simulink model "mambo_offline_simulator"  (R2022b)
settings: Solver=VariableStepAuto  StartTime=0.0  StopTime=45  RelTol=1e-3
values from neighbouring files (symbols this model uses):
  A_angles = sysd_angles.den    [parrot_mambo_main.m]
  A_thrust = sysd_thrust.den    [parrot_mambo_main.m]
  angle_sat = 0.22    [parrot_mambo_main.m]
  B_angles = sysd_angles.num    [parrot_mambo_main.m]
  B_thrust = sysd_thrust.num    [parrot_mambo_main.m]
  delay = 0.08    [parrot_mambo_main.m]
  g = 9.81    [parrot_mambo_main.m]
  GLOBAL_PARAMETERS = [Ts m g Kv]    [parrot_mambo_main.m]
  initial_pos_conditions_M1 = [0 0 0]    [parrot_mambo_main.m]
  K_gain_lin = lqr(A, B, Q_gain_lin, R_gain_lin)    [parrot_mambo_main.m]
  Ki_x = 0.04    [parrot_mambo_main.m]
  Ki_y = 0.04    [parrot_mambo_main.m]
  Ki_z = 0.023    [parrot_mambo_main.m]
  m = 0.075    [parrot_mambo_main.m]
  phi_biais = 0.005    [parrot_mambo_main.m]
  sat_z = 1    [parrot_mambo_main.m]
  theta_biais = 0.005    [parrot_mambo_main.m]
  Tmax = 1.0088    [parrot_mambo_main.m]
  Tmin = 0.4786    [parrot_mambo_main.m]
  Ts = 0.01    [parrot_mambo_main.m]
  variance_boucle_attitude = 1e-7    (= 1e-07)    [parrot_mambo_main.m]
  variance_qualysis = 1e-6    (= 1e-06)    [parrot_mambo_main.m]
  x0 = -1.18    [parrot_mambo_main.m]
  y0 = -1.21    [parrot_mambo_main.m]
  z0 = 0.8    [parrot_mambo_main.m]
libraries: simulink x2, slpidlib x1
settings Model: Creator=susbielp  LastModifiedBy=phatdo
settings SolverCC: AlgebraicLoopSolver=TrustRegion
settings DataIOCC: ReturnWorkspaceOutputs=off
settings DebuggingCC: UnconnectedInputMsg=warning  UnconnectedOutputMsg=warning  UnconnectedLineMsg=warning  ArithmeticOperatorsInVariantConditions=warning
settings ModelReferenceCC: EnableRefExpFcnMdlSchedulingChecks=on
settings SFSimCC: CustomCodeUndefinedFunction=UseInterfaceOnly
settings RTWCC: DLArmComputeVersion=19.05

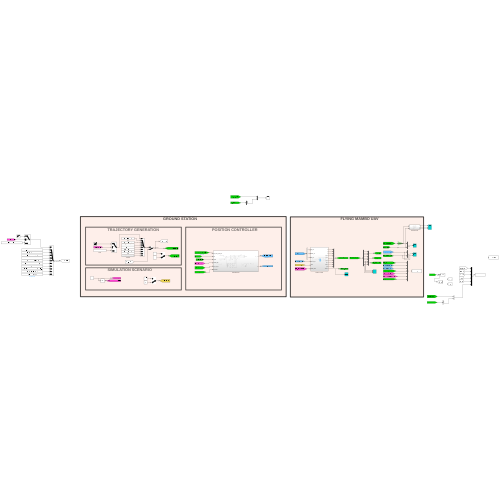
[thumbnail: Simulink's stored preview of the top-level diagram]
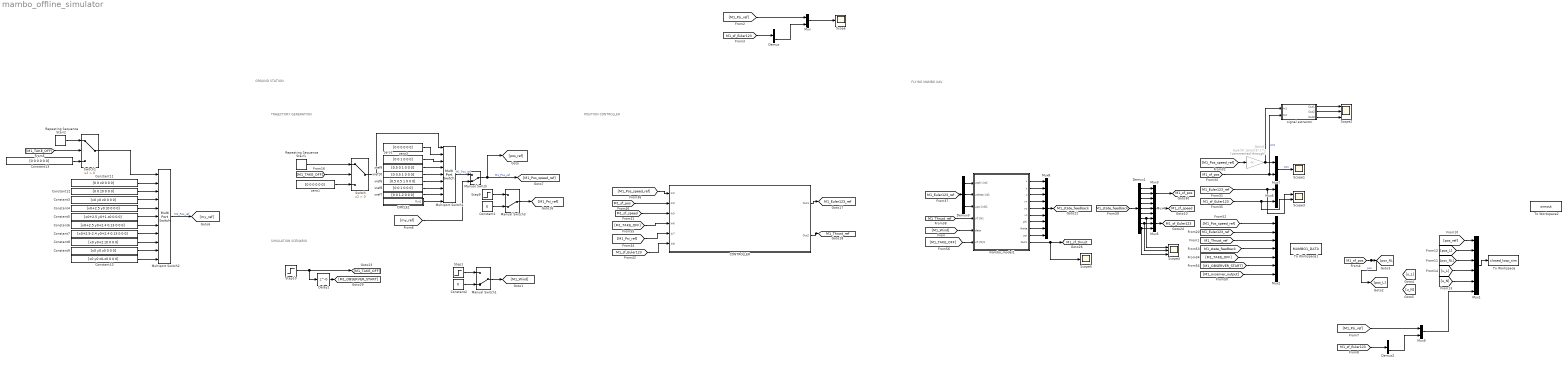
== system mambo_offline_simulator ==
  note: FLYING MAMBO UAV
  note: POSITION CONTROLLER
  note: TRAJECTORY GENERATION
  note: SIMULATION SCENARIO
  note: GROUND STATION
  CIRCLE1 : Subsystem
  CONTROLLER : Subsystem
  Constant1 : Constant  Value=0  OutDataTypeStr=double
  Constant10 : Constant  Value=[x0 y0 z0-z0 0 0 0]
  Constant11 : Constant  Value=[0 0 z0 0 0 0]
  Constant12 : Constant  Value=[0 0 z0 0 0 0]
  Constant13 : Constant  Value=[0 0 0 0 0 0]
  Constant2 : Constant  Value=0  OutDataTypeStr=double
  Constant3 : Constant  Value=[x0 y0 z0 0 0 0]
  Constant4 : Constant  Value=[x0+2.5 y0 z0 0 0 0]
  Constant5 : Constant  Value=[x0+2.5 y0+1 z0 0 0 0]
  Constant6 : Constant  Value=[x0+2.5 y0+2.4 0.13 0 0 0]
  Constant7 : Constant  Value=[x0+2.5-2.4 y0+2.4 0.13 0 0 0]
  Constant8 : Constant  Value=[x0 y0+2 z0 0 0 0]
  Constant9 : Constant  Value=[x0 y0 z0 0 0 0]
  Delay1 : Delay  DelayLength=0
  Demux : Demux  Outputs=3
  Demux1 : Demux  Outputs=9
  Demux2 : Demux  Outputs=3
  Demux3 : Demux  Outputs=3
  Gain4 : Gain  Commented=through  Gain=[eye(3) zeros(3) ]  Multiplication=Matrix(K*u) (u vector)
  Manual Switch : ManualSwitch  CurrentSetting=0
  Manual Switch1 : ManualSwitch  CurrentSetting=0
  Manual Switch3 : ManualSwitch  CurrentSetting=0
  Multiport Switch1 : MultiPortSwitch  DataPortOrder=Zero-based contiguous  Inputs=8  zeroidx=on  SaturateOnIntegerOverflow=off  InputSameDT=off
  Multiport Switch2 : MultiPortSwitch  DataPortOrder=Zero-based contiguous  Inputs=10  zeroidx=on  SaturateOnIntegerOverflow=off  InputSameDT=off
  Mux{,6..7,9} (4 alike) : Mux  Inputs=2
  Mux1 : Mux  Inputs=6
  Mux2 : Mux  Inputs=7
  Mux3 : Mux  Inputs=3
  Mux4 : Mux  Inputs=3
  Mux5 : Mux  Inputs=3
  Mux8 : Mux  Inputs=9
  Repeating Sequence Stair1 : simulink/Sources/Repeating Sequence Stair  OutValues=[1 2 1 3 1 4 1 6 7].'  tsamp=10  OutMin=[]  OutMax=[]  OutDataTypeStr=double  OutputDataTypeScalingMode=double  OutDataType=fixdt(0,8)  ConRadixGroup=Best Precision: Vector-wise  OutScaling=2^-12
  Repeating Sequence Stair2 : simulink/Sources/Repeating Sequence Stair  OutValues=[1 2 3 4 5 6 7 8 9].'  tsamp=task_ped  OutMin=[]  OutMax=[]  OutDataTypeStr=double  OutputDataTypeScalingMode=double  OutDataType=fixdt(0,8)  ConRadixGroup=Best Precision: Vector-wise  OutScaling=2^-12
  Scope : Scope
  Scope1 : Scope
  Scope2 : Scope  NumInputPorts=3
  Scope3 : Scope  NumInputPorts=2
  Scope4 : Scope  NumInputPorts=3
  Scope5 : Scope
  Step1 : Step  Time=20  Before=[0 0 0]  After=[2 0 0]  SampleTime=0
  Step10 : Step  Time=2  SampleTime=0
  Step9 : Step  Time=25  After=pi/2  SampleTime=0
  Switch : Switch  Criteria=u2 > Threshold  SaturateOnIntegerOverflow=off  InputSameDT=off
  Switch1 : Switch  Criteria=u2 > Threshold  SaturateOnIntegerOverflow=off  InputSameDT=off
  To Workspace : ToWorkspace  VariableName=closed_loop_sim  SaveFormat=Timeseries  SampleTime=-1
  To Workspace1 : ToWorkspace  VariableName=MAMBO1_DATA  SaveFormat=Timeseries  SampleTime=-1
  To Workspace2 : ToWorkspace  VariableName=simout  SaveFormat=Timeseries  SampleTime=-1
  mambo_model1 : Subsystem
  signal extractor : Subsystem
  xref10 : Constant  Value=[0 0.5 1 0 0 0]  OutDataTypeStr=double
  xref6 : Constant  Value=[0.5 0.5 1 0 0 0]  OutDataTypeStr=double
  xref7 : Constant  Value=[0 0 1.2 0 0 0]  OutDataTypeStr=double
  xref8 : Constant  Value=[0 0 1 0 0 0]  OutDataTypeStr=double
  xref9 : Constant  Value=[0.5 0 1 0 0 0]  OutDataTypeStr=double
  zero1 : Constant  Value=[0 0 0 0 0 0]  OutDataTypeStr=double
  zero2 : Constant  Value=[0 0 1 0 0 0]  OutDataTypeStr=double
  zero3 : Constant  Value=[0 0 0 0 0 0]  OutDataTypeStr=double
  tag scope: M1_Euler123_ref=global, M1_Thrust_ref=global, M1_sf_Euler123=global, M1_sf_pos=global, M1_sf_speed=global, M1_sf_thrust=global, M1_state_feedback=global
  wires:
  Mux5/1 -> [M1_sf_Euler123]
  Demux1/4 -> Mux4/1
  Demux1/1 -> Mux3/1
  Demux1/3 -> Mux3/3
  [M1_sf_pos] -> signal extractor/2(In2), Mux7/2  "pos"
  Mux7/1 -> Scope1/1  "pos"
  Demux1/6 -> Mux4/3
  [M1_OBSERVER_START] -> Mux2/6
  Demux1/5 -> Mux4/2
  [M1_sf_Euler123] -> Scope3/2, Mux6/2
  [M1_sf_speed] -> CONTROLLER/3(In5)
  [M1_Pos_speed_ref] -> CONTROLLER/1(In2)
  Demux1/2 -> Mux3/2
  Demux1/8 -> Scope4/2, Mux5/2
  Mux4/1 -> [M1_sf_speed]
  [M1_sf_pos] -> CONTROLLER/2(In3)
  [M1_Euler123_ref] -> Scope3/1, Mux6/1
  [M1_ovserver_output] -> Mux2/7
  [M1_Pos_speed_ref] -> Gain4/1
  [M1_TAKE_OFF] -> Mux2/5
  [M1_TAKE_OFF] -> CONTROLLER/4(In6)
  [M1_Euler123_ref] -> Mux2/2
  [M1_state_feedback] -> Demux1/1
  [M1_state_feedback] -> Mux2/4
  CONTROLLER/2(Out2) -> [M1_Thrust_ref]
  Mux3/1 -> [M1_sf_pos]
  CONTROLLER/1(Out1) -> [M1_Euler123_ref]
  Demux1/9 -> Scope4/3, Mux5/3
  [M1_Pos_speed_ref] -> Mux2/1
  Step10/1 -> Delay1/1, [M1_TAKE_OFF]
  Delay1/1 -> [M1_OBSERVER_START]
  CIRCLE1/1(Out1) -> Multiport Switch1/9
  zero3/1 -> Multiport Switch1/2
  Manual Switch/1 -> [pos_ref], [M1_Pos_speed_ref]  "M1_Pos_ref"
  xref8/1 -> Multiport Switch1/7
  xref7/1 -> Multiport Switch1/8
  xref9/1 -> Multiport Switch1/4
  xref10/1 -> Multiport Switch1/5
  zero2/1 -> Multiport Switch1/3
  xref6/1 -> Multiport Switch1/6
  Step9/1 -> Manual Switch3/1
  [M1_Thrust_ref] -> Mux2/3
  Manual Switch3/1 -> [M1_Psi_ref]
  Switch/1 -> Multiport Switch1/1
  [M1_TAKE_OFF] -> Switch/2
  zero1/1 -> Switch/3
  Repeating Sequence Stair1/1 -> Switch/1
  Constant1/1 -> Manual Switch3/2
  [M1_Euler123_ref] -> Demux3/1
  mambo_model1/6(vz) -> Mux8/6
  mambo_model1/8(theta) -> Mux8/8
  mambo_model1/7(phi) -> Mux8/7
  mambo_model1/5(vy) -> Mux8/5
  mambo_model1/9(psi) -> Mux8/9
  [M1_Thrust_ref] -> mambo_model1/4(uT [N])
  mambo_model1/4(vx) -> Mux8/4
  Demux3/2 -> mambo_model1/2(utheta [rd])
  Mux8/1 -> [M1_state_feedback]
  mambo_model1/10(Out1) -> Scope5/1, [M1_sf_thrust]
  mambo_model1/3(z) -> Mux8/3
  mambo_model1/2(y) -> Mux8/2
  Demux3/3 -> mambo_model1/3(upsi [rd]1)
  Demux3/1 -> mambo_model1/1(utphi [rd])
  [M1_TAKE_OFF] -> mambo_model1/6(uT [N]1)
  mambo_model1/1(x) -> Mux8/1
  [M1_Wind] -> mambo_model1/5(data)
  Step1/1 -> Manual Switch1/1
  Constant2/1 -> Manual Switch1/2
  Manual Switch1/1 -> [M1_Wind]
  Gain4/1 -> signal extractor/1(In1), Mux7/1
  signal extractor/1(Out1) -> Scope2/1
  signal extractor/2(Out2) -> Scope2/2
  signal extractor/3(Out3) -> Scope2/3
  [M1_sf_Euler123] -> Demux/1
  [M1_Psi_ref] -> Mux/1
  Demux/3 -> Mux/2
  Mux/1 -> Scope/1
  [pos_ref] -> Mux1/1
  Mux1/1 -> To Workspace/1
  [u_N] -> Mux1/5
  [pos_L] -> Mux1/2
  [pos_NL] -> Mux1/3
  [u_L] -> Mux1/4
  [M1_sf_pos] -> [pos_L], [pos_NL]  "pos"
  Repeating Sequence Stair2/1 -> Switch1/1
  [M1_TAKE_OFF] -> Switch1/2
  Switch1/1 -> Multiport Switch2/1
  Constant11/1 -> Multiport Switch2/2
  Constant13/1 -> Switch1/3
  Constant12/1 -> Multiport Switch2/3
  Multiport Switch1/1 -> Manual Switch/1  "M1_Pos_ref"
  Constant3/1 -> Multiport Switch2/4
  Constant4/1 -> Multiport Switch2/5
  Constant5/1 -> Multiport Switch2/6
  Constant6/1 -> Multiport Switch2/7
  Constant7/1 -> Multiport Switch2/8
  Constant8/1 -> Multiport Switch2/9
  Constant9/1 -> Multiport Switch2/10
  Multiport Switch2/1 -> [my_ref]  "M1_Pos_ref"
  [my_ref] -> Manual Switch/2
  [M1_Psi_ref] -> CONTROLLER/5(In7)
  [M1_sf_Euler123] -> CONTROLLER/6(In8)
  [M1_sf_Euler123] -> Demux2/1
  [M1_Psi_ref] -> Mux9/1
  Demux2/3 -> Mux9/2
  Mux9/1 -> Mux1/6
  Demux1/7 -> Scope4/1, Mux5/1
  Constant10/1 -> Multiport Switch2/11

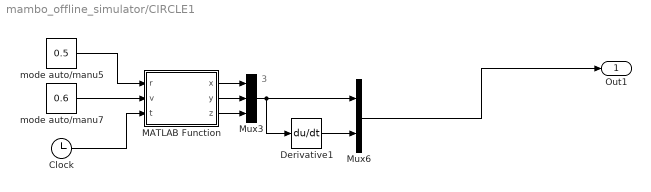
== system mambo_offline_simulator/CIRCLE1 ==
  note: 3
  Clock : Clock
  Derivative1 : Derivative  CoefficientInTFapproximation=4*Ts
  MATLAB Function : MATLAB Function  TreatAsAtomicUnit=on
  Mux3 : Mux  Inputs=3
  Mux6 : Mux  Inputs=2
  mode auto/manu5 : Constant  Value=0.5  OutDataTypeStr=double
  mode auto/manu7 : Constant  Value=0.6  OutDataTypeStr=double
  Out1 : Outport
  wires:
  MATLAB Function/2(y) -> Mux3/2
  Derivative1/1 -> Mux6/2
  Mux3/1 -> Mux6/1, Derivative1/1
  Mux6/1 -> Out1/1
  mode auto/manu5/1 -> MATLAB Function/1(r)
  Clock/1 -> MATLAB Function/3(t)
  MATLAB Function/1(x) -> Mux3/1
  mode auto/manu7/1 -> MATLAB Function/2(v)
  MATLAB Function/3(z) -> Mux3/3

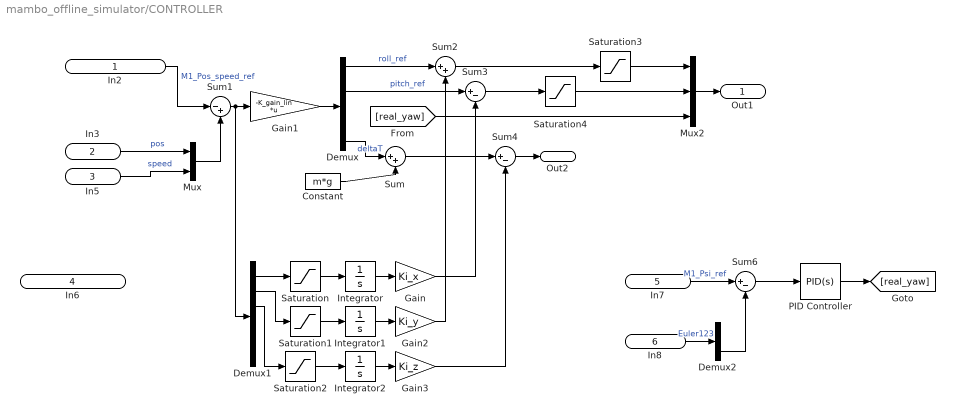
== system mambo_offline_simulator/CONTROLLER ==
  In2 : Inport
  In3 : Inport  Port=2
  In5 : Inport  Port=3
  In6 : Inport  Port=4
  In7 : Inport  Port=5
  In8 : Inport  Port=6
  Constant : Constant  Value=m*g
  Demux : Demux
  Demux1 : Demux  Outputs=6
  Demux2 : Demux  Outputs=3
  Gain : Gain  Gain=Ki_x
  Gain1 : Gain  Gain=-K_gain_lin  Multiplication=Matrix(K*u) (u vector)
  Gain2 : Gain  Gain=Ki_y
  Gain3 : Gain  Gain=Ki_z
  Integrator : Integrator
  Integrator1 : Integrator
  Integrator2 : Integrator
  Mux : Mux  Inputs=2
  Mux2 : Mux  Inputs=3
  PID Controller : slpidlib/PID Controller  Controller=PID  Form=Parallel  TimeDomain=Continuous-time  UseExternalTs=off  SampleTime=-1  IntegratorMethod=Forward Euler  FilterMethod=Forward Euler  ControllerParametersSource=internal  P=1.9  I=4.5  UseKiTs=off  D=0.05  N=8.8  UseFilter=on  TunerSelectOption=Transfer Function Based (PID Tuner App)  InitialConditionSource=internal  InitialConditionForIntegrator=0  InitialConditionForFilter=0  DifferentiatorICPrevScaledInput=0  ExternalReset=none  TrackingMode=off  Kt=1  LimitOutput=off  SatLimitsSource=internal  UpperSaturationLimit=inf  LowerSaturationLimit=-inf  LinearizeAsGain=on  AntiWindupMode=none  Kb=1  LimitIntegrator=off  UpperIntegratorSaturationLimit=inf  LowerIntegratorSaturationLimit=-inf  POutMin=[]  POutMax=[]  IOutMin=[]  IOutMax=[]  DOutMin=[]  DOutMax=[]  NOutMin=[]  NOutMax=[]  SumOutMin=[]  SumOutMax=[]  SaturationOutMin=[]  SaturationOutMax=[]  PParamMin=[]  PParamMax=[]  IParamMin=[]  IParamMax=[]  DParamMin=[]  DParamMax=[]  NParamMin=[]  NParamMax=[]  KbParamMin=[]  KbParamMax=[]  KtParamMin=[]  KtParamMax=[]  KbOutMin=[]  KbOutMax=[]  KtOutMin=[]  KtOutMax=[]  IntegratorOutMin=[]  IntegratorOutMax=[]  FilterOutMin=[]  FilterOutMax=[]  SumI1OutMin=[]  SumI1OutMax=[]  SumI2OutMin=[]  SumI2OutMax=[]  SumI3OutMin=[]  SumI3OutMax=[]  SumI4OutMin=[]  SumI4OutMax=[]  SumDOutMin=[]  SumDOutMax=[]  DifferentiatorOutMin=[]  DifferentiatorOutMax=[]  FilterDiffOutCoefMin=[]  FilterDiffOutCoefMax=[]  ReciprocalOutMin=[]  ReciprocalOutMax=[]  SumDenOutMin=[]  SumDenOutMax=[]  SumNumOutMin=[]  SumNumOutMax=[]  DivideOutMin=[]  DivideOutMax=[]  UdiffTsProdOutMin=[]  UdiffTsProdOutMax=[]  NTsProdOutMin=[]  NTsProdOutMax=[]  UintegralTsProdOutMin=[]  UintegralTsProdOutMax=[]  UngainTsProdOutMin=[]  UngainTsProdOutMax=[]  ClampingZeroOutDataTypeStr=Inherit: Inherit via back propagation  ClampingZeroOutMin=[]  ClampingZeroOutMax=[]  FilterDenConstantOutDataTypeStr=Inherit: Inherit via back propagation  FilterDenConstantOutMin=[]  FilterDenConstantOutMax=[]  PCopyOutDataTypeStr=Inherit: Inherit via back propagation  PCopyOutMin=[]  PCopyOutMax=[]  NCopyOutDataTypeStr=Inherit: Inherit via back propagation  NCopyOutMin=[]  NCopyOutMax=[]  IntegratorContinuousStateAttributes=''  IntegratorStateMustResolveToSignalObject=off  IntegratorRTWStateStorageClass=Auto  FilterContinuousStateAttributes=''  FilterStateMustResolveToSignalObject=off  FilterRTWStateStorageClass=Auto  ParallelPVariant=InternalParameters  IdealPVariant=Disabled  IVariant=InternalParameters  DVariant=InternalParameters  IntegratorVariant=Continuous  SatVariant=Disabled  AWVariant=Passthrough  PCopyVariant=Disabled  TRVariant=Disabled  FdbkBlocksVariant=Forward  IdealPFdbkVariant=Disabled  SatFdbkVariant=Disabled  DerivativeFilterVariant=ContFilter  NVariant=InternalParameters  NCopyVariant=Disabled  FilterICVariant=InternalICsFilter  IntegratorICVariant=InternalICs  ExternalResetVariant=Disabled  TRSumVariant=Passthrough  SumFdbkVariant=Disabled  SumVariant=Sum_PID  TsampFilterVariant=InternalTs  TsampNgainVariant=Passthrough  TsampIntegralVariant=Passthrough  ExternalSaturationOutDataTypeStr=Inherit: Same as second input
  Saturation : Saturate  UpperLimit=0.02  LowerLimit=-0.02
  Saturation1 : Saturate  UpperLimit=0.02  LowerLimit=-0.02
  Saturation2 : Saturate  UpperLimit=sat_z  LowerLimit=-sat_z
  Saturation3 : Saturate  UpperLimit=0.1  LowerLimit=-0.1
  Saturation4 : Saturate  UpperLimit=0.1  LowerLimit=-0.1
  Sum : Sum  Inputs=|++
  Sum1 : Sum  Inputs=|-+
  Sum2 : Sum  Inputs=|++
  Sum3 : Sum  Inputs=|+-
  Sum4 : Sum  Inputs=|+-
  Sum6 : Sum  Inputs=|+-
  Out1 : Outport
  Out2 : Outport  Port=2
  wires:
  Sum1/1 -> Demux1/1, Gain1/1
  In2/1 -> Sum1/1  "M1_Pos_speed_ref"
  Mux/1 -> Sum1/2
  Gain1/1 -> Demux/1
  In5/1 -> Mux/2  "speed"
  Mux2/1 -> Out1/1
  Constant/1 -> Sum/2
  Demux/4 -> Sum/1  "deltaT"
  In3/1 -> Mux/1  "pos"
  Demux1/3 -> Saturation2/1
  Demux1/1 -> Saturation/1
  Demux/1 -> Sum2/1  "roll_ref"
  Sum2/1 -> Saturation3/1
  Demux/2 -> Sum3/1  "pitch_ref"
  Sum3/1 -> Saturation4/1
  Sum4/1 -> Out2/1
  Sum/1 -> Sum4/1
  Integrator2/1 -> Gain3/1
  Gain/1 -> Sum3/2
  Gain2/1 -> Sum2/2
  Integrator/1 -> Gain/1
  Integrator1/1 -> Gain2/1
  Gain3/1 -> Sum4/2
  Saturation/1 -> Integrator/1
  Saturation1/1 -> Integrator1/1
  Demux1/2 -> Saturation1/1
  [real_yaw] -> Mux2/3
  In7/1 -> Sum6/1  "M1_Psi_ref"
  In8/1 -> Demux2/1  "Euler123"
  Sum6/1 -> PID Controller/1
  Demux2/3 -> Sum6/2
  PID Controller/1 -> [real_yaw]
  Saturation2/1 -> Integrator2/1
  Saturation3/1 -> Mux2/1
  Saturation4/1 -> Mux2/2

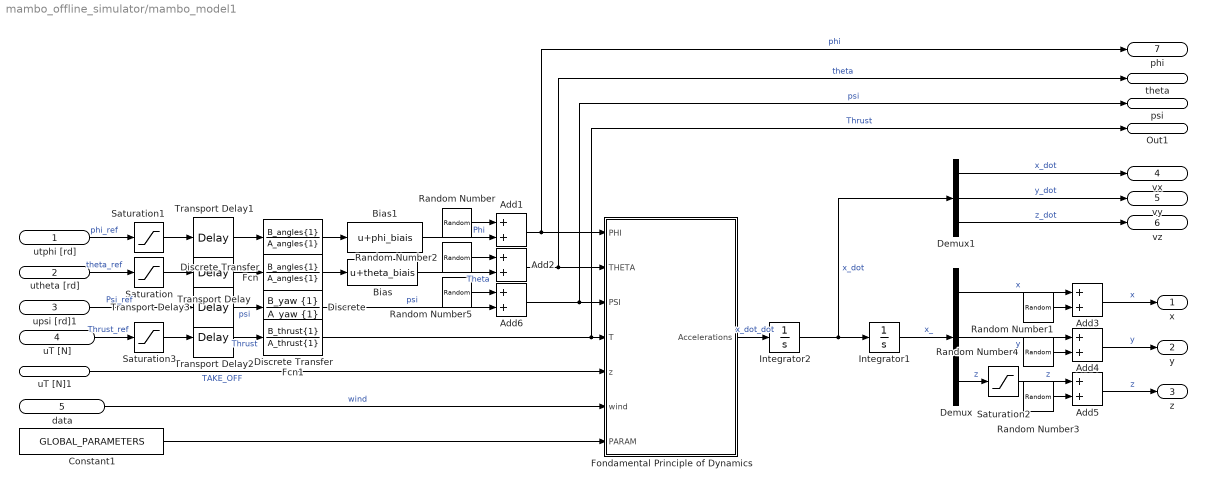
== system mambo_offline_simulator/mambo_model1 ==
  utphi [rd] : Inport
  utheta [rd] : Inport  Port=2
  upsi [rd]1 : Inport  Port=3
  uT [N] : Inport  Port=4
  data : Inport  Port=5
  uT [N]1 : Inport  Port=6
  " " : DiscreteTransferFcn  Numerator=B_angles{1}  Denominator=A_angles{1}  SampleTime=Ts
  Add{1..6} (6 alike) : Sum
  Bias : Bias  Bias=theta_biais  SaturateOnIntegerOverflow=off
  Bias1 : Bias  Bias=phi_biais  SaturateOnIntegerOverflow=off
  Constant1 : Constant  Value=GLOBAL_PARAMETERS
  Demux : Demux  Outputs=3
  Demux1 : Demux  Outputs=3
  "Discrete " : DiscreteTransferFcn  Numerator=B_yaw {1}  Denominator=A_yaw {1}  SampleTime=Ts
  Discrete Transfer Fcn : DiscreteTransferFcn  Numerator=B_angles{1}  Denominator=A_angles{1}  SampleTime=Ts
  Discrete Transfer Fcn1 : DiscreteTransferFcn  Numerator=B_thrust{1}  Denominator=A_thrust{1}  SampleTime=Ts
  Fondamental Principle of Dynamics : MATLAB Function  TreatAsAtomicUnit=on
  Integrator1 : Integrator  InitialCondition=initial_pos_conditions_M1
  Integrator2 : Integrator  InitialCondition=[0 0 0]
  Random Number : RandomNumber  Variance=variance_boucle_attitude  Seed=0.5  SampleTime=Ts
  Random Number1 : RandomNumber  Variance=variance_qualysis  Seed=10  SampleTime=Ts
  Random Number2 : RandomNumber  Variance=variance_boucle_attitude  Seed=0.5  SampleTime=Ts
  Random Number3 : RandomNumber  Variance=variance_qualysis  Seed=10  SampleTime=Ts
  Random Number4 : RandomNumber  Variance=variance_qualysis  Seed=10  SampleTime=Ts
  Random Number5 : RandomNumber  Variance=variance_boucle_attitude  Seed=0.5  SampleTime=Ts
  Saturation : Saturate  UpperLimit=angle_sat  LowerLimit=-angle_sat
  Saturation1 : Saturate  UpperLimit=angle_sat  LowerLimit=-angle_sat
  Saturation2 : Saturate  UpperLimit=inf  LowerLimit=0
  Saturation3 : Saturate  UpperLimit=Tmax  LowerLimit=Tmin
  Transport Delay{,1..3} (4 alike) : TransportDelay  DelayTime=delay
  x : Outport  VectorParamsAs1DForOutWhenUnconnected=off
  y : Outport  Port=2  VectorParamsAs1DForOutWhenUnconnected=off
  z : Outport  Port=3  VectorParamsAs1DForOutWhenUnconnected=off
  vx : Outport  Port=4  VectorParamsAs1DForOutWhenUnconnected=off
  vy : Outport  Port=5  VectorParamsAs1DForOutWhenUnconnected=off
  vz : Outport  Port=6  VectorParamsAs1DForOutWhenUnconnected=off
  phi : Outport  Port=7  VectorParamsAs1DForOutWhenUnconnected=off
  theta : Outport  Port=8  VectorParamsAs1DForOutWhenUnconnected=off
  psi : Outport  Port=9  VectorParamsAs1DForOutWhenUnconnected=off
  Out1 : Outport  Port=10
  wires:
  Transport Delay/1 -> Discrete Transfer Fcn/1
  utphi [rd]/1 -> Saturation1/1  "phi_ref"
  utheta [rd]/1 -> Saturation/1  "theta_ref"
  Saturation/1 -> Transport Delay/1
  uT [N]/1 -> Saturation3/1  "Thrust_ref"
  Demux/1 -> Add3/1  "x"
  Integrator2/1 -> Integrator1/1, Demux1/1  "x_dot"
  Transport Delay1/1 -> " "/1
  Demux1/1 -> vx/1  "x_dot"
  Fondamental Principle of Dynamics/1(Accelerations) -> Integrator2/1  "x_dot_dot"
  Saturation1/1 -> Transport Delay1/1
  " "/1 -> Bias1/1
  Discrete Transfer Fcn/1 -> Bias/1
  Transport Delay2/1 -> Discrete Transfer Fcn1/1  "Thrust"
  Demux1/3 -> vz/1  "z_dot"
  upsi [rd]1/1 -> Transport Delay3/1  "Psi_ref"
  Constant1/1 -> Fondamental Principle of Dynamics/7(PARAM)
  Demux1/2 -> vy/1  "y_dot"
  Integrator1/1 -> Demux/1  "x_"
  uT [N]1/1 -> Fondamental Principle of Dynamics/5(z)  "TAKE_OFF"
  Transport Delay3/1 -> "Discrete "/1  "psi"
  Add6/1 -> psi/1, Fondamental Principle of Dynamics/3(PSI)  "psi"
  Add1/1 -> Fondamental Principle of Dynamics/1(PHI), phi/1  "phi"
  Add2/1 -> theta/1, Fondamental Principle of Dynamics/2(THETA)  "theta"
  Add3/1 -> x/1  "x"
  Demux/2 -> Add4/1  "y"
  Add4/1 -> y/1  "y"
  Add5/1 -> z/1  "z"
  Discrete Transfer Fcn1/1 -> Out1/1, Fondamental Principle of Dynamics/4(T)  "Thrust"
  Demux/3 -> Saturation2/1  "z"
  Random Number/1 -> Add1/1
  Random Number2/1 -> Add2/1
  Random Number1/1 -> Add3/2
  Random Number4/1 -> Add4/2
  Random Number3/1 -> Add5/2
  Random Number5/1 -> Add6/1
  data/1 -> Fondamental Principle of Dynamics/6(wind)  "wind"
  Saturation3/1 -> Transport Delay2/1
  Bias1/1 -> Add1/2  "Phi"
  Bias/1 -> Add2/2  "Theta"
  "Discrete "/1 -> Add6/2  "psi"
  Saturation2/1 -> Add5/1  "z"

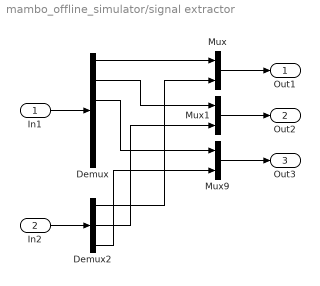
== system mambo_offline_simulator/signal extractor ==
  In1 : Inport
  In2 : Inport  Port=2
  Demux : Demux  Outputs=6
  Demux2 : Demux  Outputs=3
  Mux : Mux  Inputs=2
  Mux1 : Mux  Inputs=2
  Mux9 : Mux  Inputs=2
  Out1 : Outport
  Out2 : Outport  Port=2
  Out3 : Outport  Port=3
  wires:
  Demux/2 -> Mux1/1
  Demux2/1 -> Mux/2
  Demux/1 -> Mux/1
  Demux/3 -> Mux9/1
  Demux2/2 -> Mux1/2
  Demux2/3 -> Mux9/2
  Mux/1 -> Out1/1
  Mux1/1 -> Out2/1
  Mux9/1 -> Out3/1
  In1/1 -> Demux/1
  In2/1 -> Demux2/1

== matlab function mambo_offline_simulator/CIRCLE1/MATLAB Function ==
  data: x output; r input; y output; v input; t input; z output
function [x,y,z]= fcn(r,v,t)
w=v/r;
x=r*cos(w*t);
y=r*sin(w*t);
z=1;

== matlab function mambo_offline_simulator/mambo_model1/Fondamental Principle of Dynamics ==
  data: PHI input; Accelerations output; THETA input; PSI input; T input; z input; wind input; PARAM input
function Accelerations = fcn(PHI,THETA,PSI,T,z, wind, PARAM)

Ts = PARAM(1) ;
m = PARAM(2) ;
g = PARAM(3) ; 
Kv = PARAM(4) ;

% Rx = [1,    0    ,      0   ;...
%           0, cos(PHI), -sin(PHI);...
%           0, sin(PHI), cos(PHI)];
%   
% Ry = [ cos(THETA), 0, sin(THETA);...
%            0     , 1,      0    ;...
%       -sin(THETA), 0, cos(THETA)];
% 
% Rz = [cos(PSI), -sin(PSI), 0;...
%       sin(PSI),  cos(PSI), 0;...
%          0    ,     0    , 1];
% 
% R = Rx*(Ry*Rz);

  
% %% ------------------------------------- AUTRE ROTATION -------------------
    phi = PHI ;
    theta = THETA ;
    psi = PSI ;


    R = [ cos(theta)*cos(psi)    sin(phi)*sin(theta)*cos(psi)-cos(phi)*sin(psi)          cos(phi)*sin(theta)*cos(psi)+sin(psi)*sin(phi) ;
         cos(theta)*sin(psi)        sin(phi)*sin(theta)*sin(psi)+cos(phi)*cos(psi)        cos(phi)*sin(theta)*sin(psi)-sin(phi)*cos(psi) ;
           - sin(theta)                     sin(phi)*cos(theta)                                 cos(phi)*cos(theta) ] ;


%% ----------------------------------- ACCELERATIONS ----------------------
Accelerations = -(1)*[0 0 g]' + (1/m)*R*[0 0 T]';

% if TAKE_OFF ~=1 
%     Accelerations = [0 0 0]' ;
% else
%     Accelerations = -(1)*[0 0 g]' + (1/m)*R*[0 0 T]';
% end
if z <= 0. 
    Accelerations = [0 0 0]' ;
else
    Accelerations = -(1)*[0 0 g]' + (1/m)*R*[0 0 T]' + (1/m)*Kv*norm(wind)*wind ;
end
% Accelerations =  R*[0 0 T]';

% Accelerations = -(1)*[0 0 g]' + (1/m)*R*[0 0 T]';
end
